simulink model "pwmoutput_task"  (Simulink 3.00)
libraries: mathlib x5, genlib x2, arclib x1

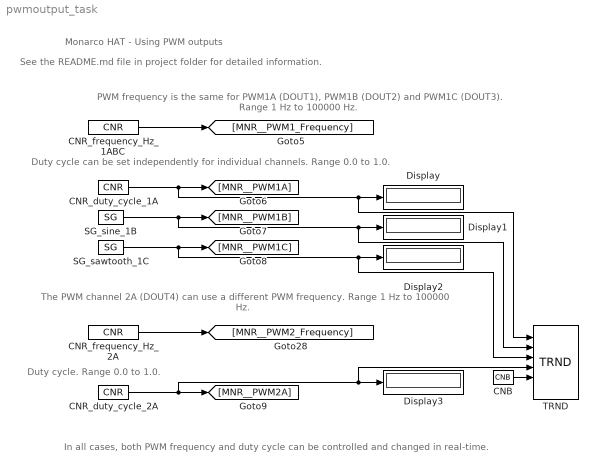
== system pwmoutput_task ==
  note: See the README.md file in project folder for detailed information.
  note: Monarco HAT - Using PWM outputs
  note: In all cases, both PWM frequency and duty cycle can be controlled and changed in real-time.
  note: PWM frequency is the same for PWM1A (DOUT1), PWM1B (DOUT2) and PWM1C (DOUT3). Range 1 Hz to 100000 Hz.
  note: Duty cycle can be set independently for individual channels. Range 0.0 to 1.0.
  note: Duty cycle. Range 0.0 to 1.0.
  note: The PWM channel 2A (DOUT4) can use a different PWM frequency. Range 1 Hz to 100000 Hz.
  CNB : mathlib/CNB  YCN=on
  CNR_duty_cycle_1A : mathlib/CNR  ycn=0.33
  CNR_duty_cycle_2A : mathlib/CNR  ycn=0.5
  CNR_frequency_Hz_1ABC : mathlib/CNR  ycn=5000
  CNR_frequency_Hz_2A : mathlib/CNR  ycn=10
  Display{,1..3} (4 alike) : Display
      settings: Format=short
  SG_sawtooth_1C : genlib/SG  isig=3: SAWTOOTH  amp=0.5  freq=0.333  phase=0  offset=0.5  ifrunit=1: Hz  iphunit=1: degrees
  SG_sine_1B : genlib/SG  isig=1: SINE  amp=0.5  freq=0.1  phase=0  offset=0.5  ifrunit=1: Hz  iphunit=1: degrees
  TRND : arclib/TRND  n=4  l=5000  btype=8: Double  ptype1=1: Store  ptype2=1: Store  ptype3=1: Store  ptype4=1: Store  pfac=1  afac=0  arc=0  id=0  Title=Duty cycles of PWM outputs  timesrc=1: CORETIMER
  wires:
  CNB/1 -> TRND/5
  CNR_duty_cycle_1A/1 -> [MNR__PWM1A], Display/1, TRND/1
  CNR_duty_cycle_2A/1 -> [MNR__PWM2A], Display3/1, TRND/4
  CNR_frequency_Hz_1ABC/1 -> [MNR__PWM1_Frequency]
  CNR_frequency_Hz_2A/1 -> [MNR__PWM2_Frequency]
  SG_sawtooth_1C/1 -> [MNR__PWM1C], Display2/1, TRND/3
  SG_sine_1B/1 -> [MNR__PWM1B], Display1/1, TRND/2
